simulink subsystem "mbd_example_nvmem_test"  (R2022b)
settings: Solver=VariableStepAuto  StartTime=0.0  StopTime=10.0  RelTol=1e-3
values from neighbouring files (symbols this model uses):
  NVMEM_DATA_ADDRESS = 0x807F800    [mbd_example_nvmem_init.m]
  T_s_LED2 = 1/LED2_Hz    (= 1)    [mbd_example_nvmem_init.m]
libraries: MbdLib_PortalDiag x10, MbdLib_Nvmem x5
settings Model: Creator=KenYoshioka  LastModifiedBy=KenYoshioka

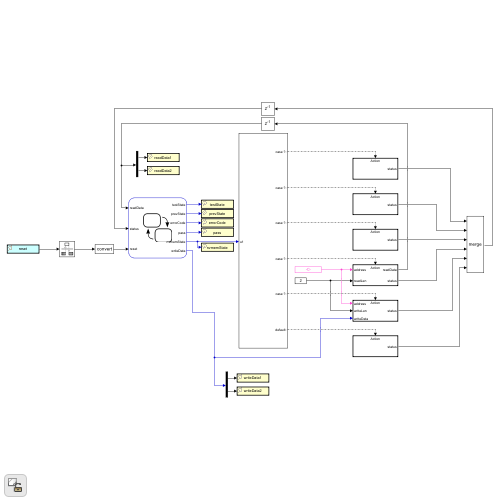
[thumbnail: Simulink's stored preview of the top-level diagram]
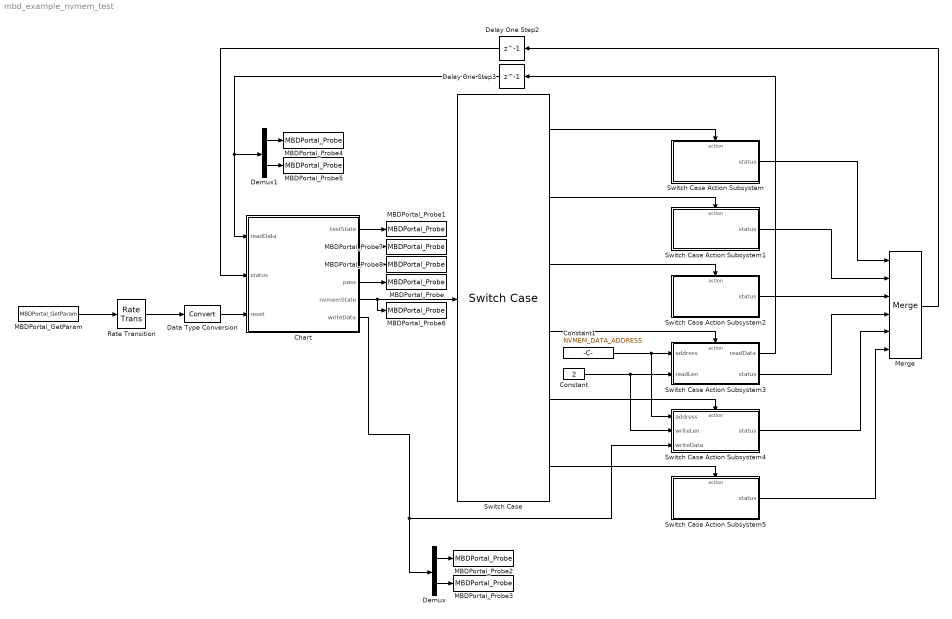
== system mbd_example_nvmem_test ==
  Chart : Stateflow chart  TreatAsAtomicUnit=on  SystemSampleTime=T_s_LED2
      settings: PortSchema="{\"entries\":[{\"content\":{\"sides\":[{\"content\":{\"connectorIds\":[\"In2\",\"In1\",\"In3\"]},\"type\":\"ConnectorPlacement.EquallySpacedRectSide\",\"uuid\":\"b4f13df6-641b-4caf-935e-2575d012ed0a\"},{\"content\":{\"connectorIds\":[\"Out4\",\"Out5\",\"Out6\",\"Out3\",\"Out1\",\"Out2\"],\"side\":\"RIGHT\"},\"type\":\"ConnectorPlacement.EquallySpacedRectSide\",\"uuid\":\"680411e5-570a-4ed3-9978-f5588f536136\"},{\"content\":{\"connectorIds\":[],\"side\":\"TOP\"},\"type\":\"ConnectorPlacement.EquallySpacedRectSide\",\"uuid\":\"d2289b2e-cf90-400d-b288-547edde60e25\"}]},\"type\":\"ConnectorPlacement.EquallySpacedConnector\",\"uuid\":\"6e9a1aa8-0192-41a2-aff8-19ffc4f986fd\"}],\"packageUris\":[\"http://schema.mathworks.com/mf0/Connector/R2020b\"],\"version\":\"1.0\"}"
  Constant : Constant  Value=2  OutDataTypeStr=uint32
  Constant1 : Constant  Value=NVMEM_DATA_ADDRESS  OutDataTypeStr=uint32
  Data Type Conversion : DataTypeConversion  SaturateOnIntegerOverflow=off  RndMeth=Floor
  Delay One Step2 : Delay  DelayLength=1
  Delay One Step3 : Delay  DelayLength=1
  Demux : Demux  Outputs=2
  Demux1 : Demux  Outputs=2
  MBDPortal_GetParam : MbdLib_PortalDiag/MBDPortal_GetParam  Param_ParamName=reset  Param_ParamDefault=0  Param_ParamIndex=0  Param_ParamMax=MBDPortal_ParamNum
      settings: SourceProductName=Peloton Component Library
  MBDPortal_Probe : MbdLib_PortalDiag/MBDPortal_Probe  Param_SigNameInherited=on  Param_SigName=pass  Param_SigIndex=0  Param_SigMax=MBDPortal_SignalNum  Param_SampleTime=MBDPortal_CommonSampleRate
      settings: SourceProductName=Peloton Component Library
  MBDPortal_Probe1 : MbdLib_PortalDiag/MBDPortal_Probe  Param_SigNameInherited=on  Param_SigName=testState  Param_SigIndex=0  Param_SigMax=MBDPortal_SignalNum  Param_SampleTime=MBDPortal_CommonSampleRate
      settings: SourceProductName=Peloton Component Library
  MBDPortal_Probe2 : MbdLib_PortalDiag/MBDPortal_Probe  Param_SigNameInherited=on  Param_SigName=writeData1  Param_SigIndex=0  Param_SigMax=MBDPortal_SignalNum  Param_SampleTime=MBDPortal_CommonSampleRate
      settings: SourceProductName=Peloton Component Library
  MBDPortal_Probe3 : MbdLib_PortalDiag/MBDPortal_Probe  Param_SigNameInherited=on  Param_SigName=writeData2  Param_SigIndex=0  Param_SigMax=MBDPortal_SignalNum  Param_SampleTime=MBDPortal_CommonSampleRate
      settings: SourceProductName=Peloton Component Library
  MBDPortal_Probe4 : MbdLib_PortalDiag/MBDPortal_Probe  Param_SigNameInherited=on  Param_SigName=readData1  Param_SigIndex=0  Param_SigMax=MBDPortal_SignalNum  Param_SampleTime=MBDPortal_CommonSampleRate
      settings: SourceProductName=Peloton Component Library
  MBDPortal_Probe5 : MbdLib_PortalDiag/MBDPortal_Probe  Param_SigNameInherited=on  Param_SigName=readData2  Param_SigIndex=0  Param_SigMax=MBDPortal_SignalNum  Param_SampleTime=MBDPortal_CommonSampleRate
      settings: SourceProductName=Peloton Component Library
  MBDPortal_Probe6 : MbdLib_PortalDiag/MBDPortal_Probe  Param_SigNameInherited=on  Param_SigName=nvmemState  Param_SigIndex=0  Param_SigMax=MBDPortal_SignalNum  Param_SampleTime=MBDPortal_CommonSampleRate
      settings: SourceProductName=Peloton Component Library
  MBDPortal_Probe7 : MbdLib_PortalDiag/MBDPortal_Probe  Param_SigNameInherited=on  Param_SigName=prevState  Param_SigIndex=0  Param_SigMax=MBDPortal_SignalNum  Param_SampleTime=MBDPortal_CommonSampleRate
      settings: SourceProductName=Peloton Component Library
  MBDPortal_Probe8 : MbdLib_PortalDiag/MBDPortal_Probe  Param_SigNameInherited=on  Param_SigName=errorCode  Param_SigIndex=0  Param_SigMax=MBDPortal_SignalNum  Param_SampleTime=MBDPortal_CommonSampleRate
      settings: SourceProductName=Peloton Component Library
  Merge : Merge  Inputs=6
  Rate Transition : RateTransition
  Switch Case : SwitchCase  CaseConditions={NVMEM_E.UNLOCK,NVMEM_E.LOCK,NVMEM_E.ERASE,NVMEM_E.READ,NVMEM_E.WRITE}
  Switch Case Action Subsystem : Subsystem  TreatAsAtomicUnit=on
  Switch Case Action Subsystem1 : Subsystem  TreatAsAtomicUnit=on
  Switch Case Action Subsystem2 : Subsystem  TreatAsAtomicUnit=on
  Switch Case Action Subsystem3 : Subsystem  TreatAsAtomicUnit=on
  Switch Case Action Subsystem4 : Subsystem  TreatAsAtomicUnit=on
  Switch Case Action Subsystem5 : Subsystem  TreatAsAtomicUnit=on
  wires:
  Constant/1 -> Switch Case Action Subsystem3/2(readLen), Switch Case Action Subsystem4/2(writeLen)
  Chart/4(testState) -> MBDPortal_Probe1/1
  Chart/2(writeData) -> Switch Case Action Subsystem4/3(writeData), Demux/1
  Constant1/1 -> Switch Case Action Subsystem3/1(address), Switch Case Action Subsystem4/1(address)
  Demux1/2 -> MBDPortal_Probe5/1
  Demux/2 -> MBDPortal_Probe3/1
  Switch Case/3 -> Switch Case Action Subsystem2/Action
  Delay One Step3/1 -> Chart/2(readData), Demux1/1
  Switch Case/6 -> Switch Case Action Subsystem5/Action
  Rate Transition/1 -> Data Type Conversion/1
  Merge/1 -> Delay One Step2/1
  Delay One Step2/1 -> Chart/1(status)
  Switch Case/1 -> Switch Case Action Subsystem/Action
  Switch Case Action Subsystem4/1(status) -> Merge/5
  Data Type Conversion/1 -> Chart/3(reset)
  Switch Case Action Subsystem/1(status) -> Merge/1
  Demux/1 -> MBDPortal_Probe2/1
  Switch Case Action Subsystem5/1(status) -> Merge/6
  Chart/1(nvmemState) -> Switch Case/1, MBDPortal_Probe6/1
  MBDPortal_GetParam/1 -> Rate Transition/1
  Switch Case Action Subsystem1/1(status) -> Merge/2
  Switch Case Action Subsystem3/2(status) -> Merge/4
  Demux1/1 -> MBDPortal_Probe4/1
  Switch Case/2 -> Switch Case Action Subsystem1/Action
  Switch Case/4 -> Switch Case Action Subsystem3/Action
  Switch Case Action Subsystem2/1(status) -> Merge/3
  Chart/3(pass) -> MBDPortal_Probe/1
  Chart/5(prevState) -> MBDPortal_Probe7/1
  Chart/6(errorCode) -> MBDPortal_Probe8/1
  Switch Case Action Subsystem3/1(readData) -> Delay One Step3/1
  Switch Case/5 -> Switch Case Action Subsystem4/Action

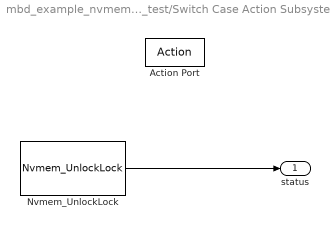
== system mbd_example_nvmem_test/Switch Case Action Subsystem ==
  Action Port : ActionPort
  Nvmem_UnlockLock : MbdLib_Nvmem/Nvmem_UnlockLock  Priority=0  Param_action=Unlock  Param_priority=0  Param_sampleTime=-1
      settings: AttributesFormatString=priority=%<priority>  SourceProductName=Peloton Interface Library
  status : Outport
  wires:
  Nvmem_UnlockLock/1 -> status/1

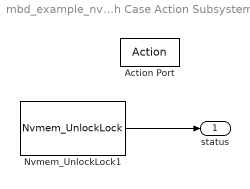
== system mbd_example_nvmem_test/Switch Case Action Subsystem1 ==
  Action Port : ActionPort
  Nvmem_UnlockLock1 : MbdLib_Nvmem/Nvmem_UnlockLock  Priority=0  Param_action=Lock  Param_priority=0  Param_sampleTime=-1
      settings: AttributesFormatString=priority=%<priority>  SourceProductName=Peloton Interface Library
  status : Outport
  wires:
  Nvmem_UnlockLock1/1 -> status/1

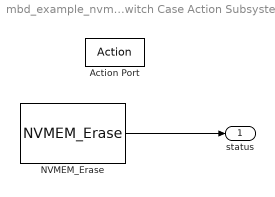
== system mbd_example_nvmem_test/Switch Case Action Subsystem2 ==
  Action Port : ActionPort
  NVMEM_Erase : MbdLib_Nvmem/NVMEM_Erase  Param_address=0  Param_type=0  Param_bank=1  Param_offset=NVMEM_ERASE_OFFSET  Param_num=1  Param_voltageRange=NVMEM_ERASE_VOLTAGE  Param_sampleTime=-1  Param_update=1
      settings: SourceProductName=Peloton Interface Library
  status : Outport
  wires:
  NVMEM_Erase/1 -> status/1

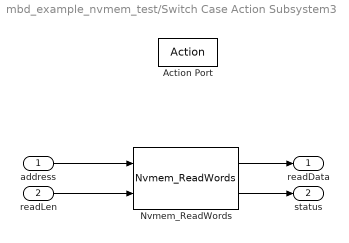
== system mbd_example_nvmem_test/Switch Case Action Subsystem3 ==
  address : Inport
  readLen : Inport  Port=2
  Action Port : ActionPort
  Nvmem_ReadWords : MbdLib_Nvmem/Nvmem_ReadWords  Param_wordLim=2  Param_sampleTime=-1
      settings: SourceProductName=Peloton Interface Library
  readData : Outport
  status : Outport  Port=2
  wires:
  Nvmem_ReadWords/2 -> status/1
  Nvmem_ReadWords/1 -> readData/1
  readLen/1 -> Nvmem_ReadWords/2
  address/1 -> Nvmem_ReadWords/1

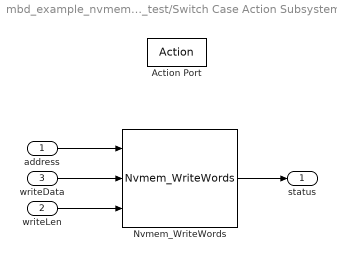
== system mbd_example_nvmem_test/Switch Case Action Subsystem4 ==
  address : Inport
  writeLen : Inport  Port=2
  writeData : Inport  Port=3
  Action Port : ActionPort
  Nvmem_WriteWords : MbdLib_Nvmem/Nvmem_WriteWords  Param_sampleTime=-1
      settings: SourceProductName=Peloton Interface Library
  status : Outport
  wires:
  writeLen/1 -> Nvmem_WriteWords/3
  writeData/1 -> Nvmem_WriteWords/2
  address/1 -> Nvmem_WriteWords/1
  Nvmem_WriteWords/1 -> status/1

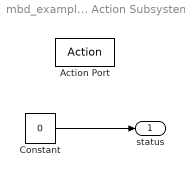
== system mbd_example_nvmem_test/Switch Case Action Subsystem5 ==
  Action Port : ActionPort
  Constant : Constant  Value=0  OutDataTypeStr=uint8
  status : Outport
  wires:
  Constant/1 -> status/1

== stateflow chart mbd_example_nvmem_test/Chart ==
  state NVMEM_TEST
    en:
    pass = false;
    state NVMEM_IN_PROGRESS
      ex:
      nvmemState = NVMEM_E.NONE;
      state UNLOCK
        testState = 1;
        nvmemState = NVMEM_E.UNLOCK;
      state ERASE
        testState = 2;
        nvmemState = NVMEM_E.ERASE;
      state VERIFY_ERASE
        testState = 3;
        nvmemState = NVMEM_E.READ;
      state WRITE
        testState = 4;
        nvmemState = NVMEM_E.WRITE;
        writeData(1) = testData1;
        writeData(2) = testData2;
      state VERIFY_WRITE
        testState = 5;
        nvmemState = NVMEM_E.READ;
      state LOCK
        testState = 6;
        nvmemState = NVMEM_E.LOCK;
      (default) -> UNLOCK
      UNLOCK -> ERASE
      ERASE -> VERIFY_ERASE
      VERIFY_ERASE -> WRITE [order 1] : [readData(1) == emptyData && ...
          | readData(2) == emptyData]
      WRITE -> VERIFY_WRITE
      VERIFY_WRITE -> LOCK [order 1] : [readData(1) == testData1 && ...
          | readData(2) == testData2]
    state VERIFY_ERASE_FAILED
      en:
      testState = 10;
    state VERIFY_WRITE_FAILED
      en:
      testState = 11;
    state ERROR
      en:
      errorCode = status;
      prevState = testState;
      testState = 12;
    state NVMEM_PASS
      en:
      testState = 7;
      pass = true;
    (default) -> NVMEM_IN_PROGRESS
    VERIFY_ERASE -> VERIFY_ERASE_FAILED [order 2]
    VERIFY_WRITE -> VERIFY_WRITE_FAILED [order 2]
    NVMEM_IN_PROGRESS -> ERROR : [status > 0]
    LOCK -> NVMEM_PASS
  NVMEM_TEST -> NVMEM_TEST : [hasChangedFrom(reset,0)]
  data: nvmemState output Enum: NVMEM_E; status input; writeData output size=2 =[uint32(0);uint32(0)]; readData input; testData1 constant uint32 =uint32(0xAABBCC); emptyData constant uint32 =uint32(0xFFFFFFFF); pass output boolean =false; reset input uint8; testState output uint8; testData2 constant uint32 =uint32(0xDDEEFF); prevState output uint8; errorCode output uint8
